simulink model "sim_link"  (R2021b)
settings: Solver=VariableStepAuto  StartTime=0.0  StopTime=300  RelTol=1e-3
undefined symbols (not defined in the file): h, SP, T, tau
settings Model: Creator=szczy  LastModifiedBy=szczy

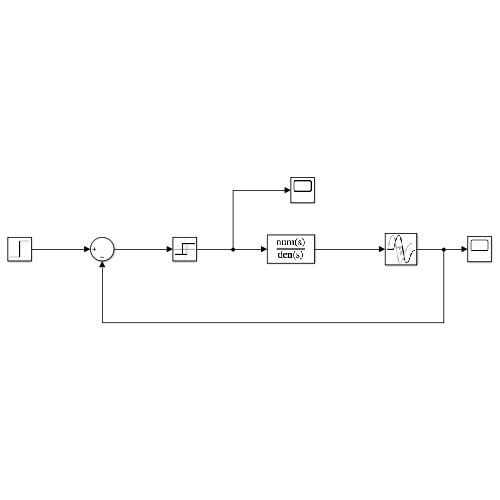
[thumbnail: Simulink's stored preview of the top-level diagram]
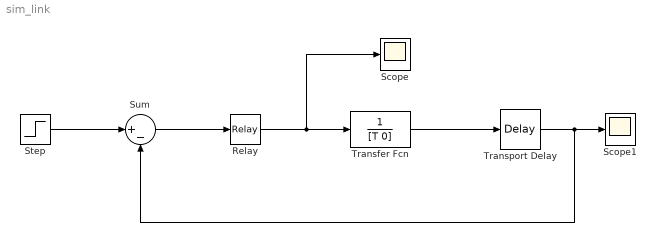
== system sim_link ==
  Relay : Relay  OnSwitchValue=h  OffSwitchValue=-h  OffOutputValue=-1
  Scope : Scope
  Scope1 : Scope
  Step : Step  After=SP  SampleTime=0
  Sum : Sum  Inputs=|+-
  Transfer Fcn : TransferFcn  Denominator=[T 0]
  Transport Delay : TransportDelay  DelayTime=tau  PadeOrder=10
  wires:
  Step/1 -> Sum/1
  Sum/1 -> Relay/1
  Relay/1 -> Scope/1, Transfer Fcn/1
  Transfer Fcn/1 -> Transport Delay/1
  Transport Delay/1 -> Sum/2, Scope1/1
